simulink model "PubIfDecisionLSM_MDL"  (R2020b)
settings: configuration reference "DspaceConfig" (kept outside this file)
PostLoadFcn:
  | if any(exist('dsrtsu_mdlpostloadfcn', 'file') ~= 0), dsrtsu_mdlpostloadfcn('Execute', bdroot); end
InitFcn:
  | , if any(exist('rtifpga_mdlclblib', 'file') ~= 0), rtifpga_mdlclblib('Init', bdroot); end,
  | , if any(exist('dsmpb_private', 'file') ~= 0), dsmpb_private('dsmpb_mdlclblib', 'Init', bdroot); end,
values from neighbouring files (symbols this model uses):
  P_LSM_ALC_Enable = 0.0    [LSM_Parameter.sldd]
  P_LSM_AwayEdge_offset = 0.1    [LSM_Parameter.sldd]
  P_LSM_CentValidErr = 1.0    [LSM_Parameter.sldd]
  P_LSM_DOP_C0_EN_Limit = 0.8    [LSM_Parameter.sldd]
  P_LSM_DOP_C0_out_Limit = 2.0    [LSM_Parameter.sldd]
  P_LSM_DOP_C1_EN_Limit : value not decoded    [LSM_Parameter.sldd]
  P_LSM_DOP_C1_out_Limit : value not decoded    [LSM_Parameter.sldd]
  P_LSM_DOP_C1AndC2_Lim_X : value not decoded    [LSM_Parameter.sldd]
  P_LSM_DOP_C2_EN_Limit : value not decoded    [LSM_Parameter.sldd]
  P_LSM_DOP_C2_out_Limit : value not decoded    [LSM_Parameter.sldd]
  P_LSM_DOP_In_Pre2Dop_Dis = 1.0    [LSM_Parameter.sldd]
  P_LSM_DOP_Out_Pre2Dop_Dis = 2.0    [LSM_Parameter.sldd]
  P_LSM_DOP_PreDis_X : value not decoded    [LSM_Parameter.sldd]
  P_LSM_DOP_PreDis_Y : value not decoded    [LSM_Parameter.sldd]
  P_LSM_DOPEnableSW = 1.0    [LSM_Parameter.sldd]
  P_LSM_DOPValid_CheckTime = 0.06    [LSM_Parameter.sldd]
  P_LSM_DoubleLine_Curr2Cent_Dislimit = 0.5    [LSM_Parameter.sldd]
  P_LSM_DoubleLine_Dop2Cent_Dislimit = 0.5    [LSM_Parameter.sldd]
  P_LSM_DoubleLine_DOPOut_C1 : value not decoded    [LSM_Parameter.sldd]
  P_LSM_DoubleLine_Pre2Cent_Dislimit = 1.0    [LSM_Parameter.sldd]
  P_LSM_Error_Limit = 0.5    [LSM_Parameter.sldd]
  P_LSM_IFV2CenterAxis = 0.0    [LSM_Parameter.sldd]
  P_LSM_IFV2RearAxis = 0.0    [LSM_Parameter.sldd]
  P_LSM_Line2Edge_limit = 0.5    [LSM_Parameter.sldd]
  P_LSM_Line_Error = 0.1    [LSM_Parameter.sldd]
  P_LSM_LineSTD_Limit = 0.15    [LSM_Parameter.sldd]
  P_LSM_NOH_Switch = 0.0    [LSM_Parameter.sldd]
  P_LSM_OTL_C0_Factor = 1.0    [LSM_Parameter.sldd]
  P_LSM_OTL_C1_Factor = 0.5    [LSM_Parameter.sldd]
  P_LSM_OTL_C2_Factor = 0.5    [LSM_Parameter.sldd]
  P_LSM_Pre2OnlyLineDis = 5.0    [LSM_Parameter.sldd]
  P_LSM_Pre_t = 0.0    [LSM_Parameter.sldd]
  P_LSM_SingleLine_Cent2Edge_Dislimit = 100.0    [LSM_Parameter.sldd]
  P_LSM_SingleLine_Curr2Cent_Dislimit = 0.2    [LSM_Parameter.sldd]
  P_LSM_SingleLine_Dop2Cent_Dislimit = 0.2    [LSM_Parameter.sldd]
  P_LSM_SingleLine_DOPOut_C1 : value not decoded    [LSM_Parameter.sldd]
  P_LSM_SingleLine_Pre2Cent_Dislimit = 0.5    [LSM_Parameter.sldd]
  P_LSM_TJALimitSpd = 60.0    [LSM_Parameter.sldd]
undefined symbols (not defined in the file or in its folder): P_lCS_IFV2CenterAxis, P_LCS_IFV2RearAxis, P_LSM_EntryEdge_offset, P_LSM_EntryLnChngEnSwitch, P_LSM_EntryVanishDis, P_LSM_LinetLostTime, P_LSM_LineWijCal_C12, P_LSM_LineWijCal_C13, P_LSM_MapValid_ErrorSwitch, P_LSM_PosLineLcFac, P_LSM_SpdLim_Stub_Spd, P_LSM_SpdLim_StubLength, P_LSM_SpdTurnAlarm
libraries: simulink x324, TrueDurationTime x11
(part 2 of 25)

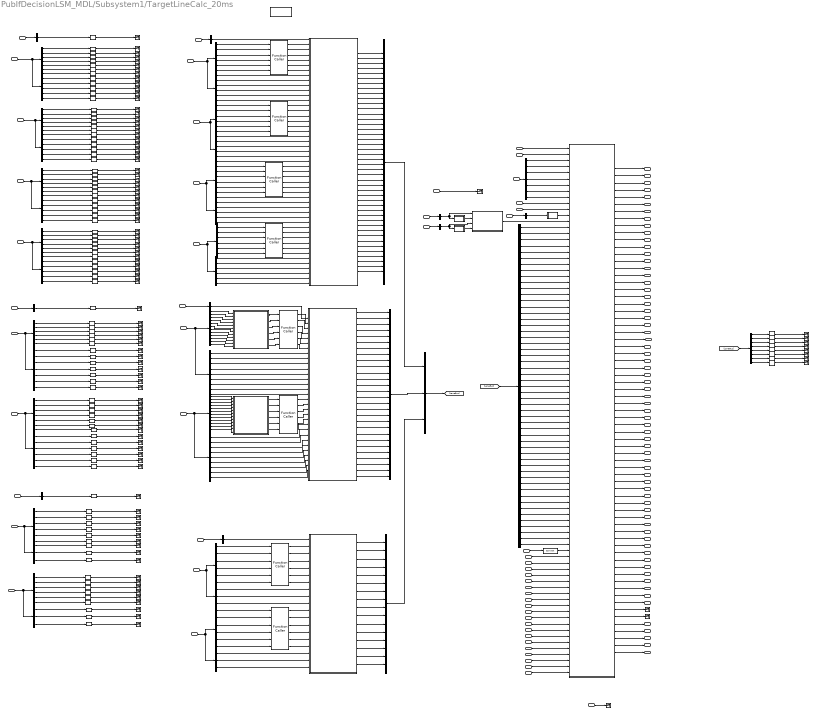
== system PubIfDecisionLSM_MDL/Subsystem1/TargetLineCalc_20ms ==
  vRef : Inport
  kap : Inport  Port=2
  EQ4_LA_ELEM_0 : Inport  Port=3
  EQ4_LA_ELEM_1 : Inport  Port=4
  EQ4_LA_ELEM_2 : Inport  Port=5
  EQ4_LA_ELEM_3 : Inport  Port=6
  LA_HDR : Inport  Port=7
  EQ4_LH_ELEM_0 : Inport  Port=8
  EQ4_LH_ELEM_1 : Inport  Port=9
  LH_HDR : Inport  Port=10
  EQ4_LRE_ELEM : Inport  Port=11
  EQ4_LRE_ELEM1 : Inport  Port=12
  LRE_HDR : Inport  Port=13
  P0TargetLine : Inport  Port=14  OutDataTypeStr=Bus: TOS_P0_TARGET_LINE_BUS
  ACCMode : Inport  Port=15
  HWASts : Inport  Port=16
  ESSSts : Inport  Port=17
  LCKSts : Inport  Port=18
  pathPredValid : Inport  Port=19
  pathPredC3 : Inport  Port=20
  pathPredC2 : Inport  Port=21
  pathPredC1 : Inport  Port=22
  pathPredC0 : Inport  Port=23
  pathPredCnt : Inport  Port=24
  PLAN_ALC_Decision : Inport  Port=25
  RFM_INTERSEC_ALERT : Inport  Port=26
  RFM_ROAD : Inport  Port=27  OutDataTypeStr=Bus: RFM_ROAD_BUS  PortDimensions=1  BusOutputAsStruct=on
  RFM_CURRENT_LANE : Inport  Port=28
  RFM_RIGHT_LANE : Inport  Port=29
  RFM_BRANCH : Inport  Port=30
  RFM_LINE_ENTRY_CL : Inport  Port=31
  RFM_LINE_EXIT_CL : Inport  Port=32
  RFM_LINE_CL : Inport  Port=33
  RFM_TSR_BUS : Inport  Port=34
  RFM_REC_LANES : Inport  Port=35
  RFM_LINE_L1 : Inport  Port=36
  RFM_LINE_R1 : Inport  Port=37
  RFM_LINE_L2 : Inport  Port=38
  RFM_LINE_R2 : Inport  Port=39
  Bus Creator : BusCreator  Inputs=44
  Bus Creator1 : BusCreator  Inputs=28
  Bus Creator2 : BusCreator  Inputs=16
  Bus Creator3 : BusCreator  Inputs=3
  Bus Selector{,1..3,25..26,32..33} (8 alike) : BusSelector  OutputSignals=LA_Line_C0,LA_Line_C1,LA_Line_C2,LA_Line_C3,LA_View_Range_Start,LA_View_Range_End
  Bus Selector10 : BusSelector  OutputSignals=LH.LeftLaneChange,LH.RightLaneChange,LA.L1Conf,LH.LH1Conf,LH.LH2Conf,LA.L4Conf,LA.L1C3,LH.LH1C3,LH.LH2C3,LA.L4C3,LA.L1C2,LH.LH1C2,LH.LH2C2,LA.L4C2,LA.L1C1,LH.LH1C1,LH.LH2C1,LA.L4C1,LA.L1C0,LH.LH1C0,LH.LH2C0,LA.L4C0,LA.L1DxMax,LH.LH1DxMax,LH.LH2DxMax,LA.L4DxMax,LA.L1Reliable,LH.LH1Reliable,LH.LH2Reliable,LA.L4Reliable,LRE.LRE1DxMax,LRE.LRE2DxMax,LRE.LRE1C3,LRE.LRE2C3,LRE.LRE1C2,LRE.LRE2C2,LRE.LRE1C1,LRE.LRE2C1,LRE.LRE1C0,LRE.LRE2C0,LRE.LRE1Conf,LRE.LRE2Conf,LRE.LRE1Reliable,LRE.LRE2Reliable,LH.LH1Type,LH.LH2Type,LH.LH1DLM,LH.LH2DLM,LH.LH1Color,LH.LH2Color,LH.LH1DECEL,LH.LH2DECEL,LA.L1Type
  Bus Selector{11..14,27..30} (8 alike) : BusSelector  OutputSignals=LA_Availability_State,LA_Lanemark_Type,LA_DLM_Type,LA_Line_Side,LA_Marker_Width,LA_Confidence
  Bus Selector15 : BusSelector  OutputSignals=LH_Availability_State,LH_Lanemark_Type,LH_DLM_Type,LH_Side,LH_Marker_Width,LH_Crossing,LH_Confidence,LH_Color,LH_DECEL_Type
  Bus Selector16 : BusSelector  OutputSignals=LH_Availability_State,LH_Lanemark_Type,LH_DLM_Type,LH_Side,LH_Marker_Width,LH_Crossing,LH_Confidence,LH_Color,LH_DECEL_Type
  Bus Selector{17..18,39..40} (4 alike) : BusSelector  OutputSignals=LRE_Availability_State,LRE_Side,LRE_Confidence
  Bus Selector19 : BusSelector  OutputSignals=LA_Adjacent_Count
  Bus Selector20 : BusSelector  OutputSignals=LA_Sync_ID
  Bus Selector21 : BusSelector  OutputSignals=LH_Sync_ID
  Bus Selector22 : BusSelector  OutputSignals=LRE_Sync_ID
  Bus Selector23 : BusSelector  OutputSignals=LH_Lanes_Count
  Bus Selector24 : BusSelector  OutputSignals=LRE_Count
  Bus Selector31 : BusSelector  OutputSignals=LA_Adjacent_Count
  Bus Selector34 : BusSelector  OutputSignals=LH_Availability_State,LH_Lanemark_Type,LH_DLM_Type,LH_Side,LH_Marker_Width,LH_Crossing,LH_Confidence
  Bus Selector35 : BusSelector  OutputSignals=LH_Availability_State,LH_Lanemark_Type,LH_DLM_Type,LH_Side,LH_Marker_Width,LH_Crossing,LH_Confidence
  Bus Selector36 : BusSelector  OutputSignals=LH_Lanes_Count
  Bus Selector37 : BusSelector  OutputSignals=LH_Line_First_C0,LH_Line_First_C1,LH_Line_First_C2,LH_Line_First_C3,LH_First_VR_Start,LH_First_VR_End
  Bus Selector38 : BusSelector  OutputSignals=LH_Line_First_C0,LH_Line_First_C1,LH_Line_First_C2,LH_Line_First_C3,LH_First_VR_Start,LH_First_VR_End
  Bus Selector4 : BusSelector  OutputSignals=LH_Line_First_C0,LH_Line_First_C1,LH_Line_First_C2,LH_Line_First_C3,LH_First_VR_Start,LH_First_VR_End,LH_Line_Second_C0,LH_Line_Second_C1,LH_Line_Second_C2,LH_Line_Second_C3,LH_Second_VR_Start,LH_Second_VR_End
  Bus Selector41 : BusSelector  OutputSignals=LRE_Count
  Bus Selector{6..7,42..43} (4 alike) : BusSelector  OutputSignals=LRE_Line_C0,LRE_Line_C1,LRE_Line_C2,LRE_Line_C3,LRE_View_Range_Start,LRE_View_Range_End
  Bus Selector5 : BusSelector  OutputSignals=LH_Line_First_C0,LH_Line_First_C1,LH_Line_First_C2,LH_Line_First_C3,LH_First_VR_Start,LH_First_VR_End,LH_Line_Second_C0,LH_Line_Second_C1,LH_Line_Second_C2,LH_Line_Second_C3,LH_Second_VR_Start,LH_Second_VR_End
  Bus Selector8 : BusSelector  OutputSignals=OTL_Valid,OTL_C3,OTL_C2,OTL_C1,OTL_C0,OTL_Range,OTL_Cnt
  Bus Selector9 : BusSelector  OutputSignals=LA.L1Conf,LA.L1DxMax,LH.LH1Conf,LH.LH1DxMax,LH.LH2Conf,LH.LH2C3,LA.L4Conf,LA.L4DxMax
  Data Type Conversion : DataTypeConversion
  DetectChange : Subsystem
  DetectChange1 : Subsystem
  DetectChange2 : Subsystem
  EQ4_LA_ELEM_4 : InportShadow  Port=3
  EQ4_LA_ELEM_5 : InportShadow  Port=4
  EQ4_LA_ELEM_6 : InportShadow  Port=5
  EQ4_LA_ELEM_7 : InportShadow  Port=6
  EQ4_LH_ELEM_2 : InportShadow  Port=9
  EQ4_LH_ELEM_3 : InportShadow  Port=8
  EQ4_LRE_ELEM2 : InportShadow  Port=12
  EQ4_LRE_ELEM3 : InportShadow  Port=11
  Function Caller{,1..7} (8 alike) : FunctionCaller  FunctionPrototype=[a0,a1,a2,a3,Rmin,Rmax] = f(A0,A1,A2,A3,Range_min,Range_max)  InputArgumentSpecifications=<Enter example>  OutputArgumentSpecifications=<Enter example>
  LALine : MATLAB Function  TreatAsAtomicUnit=on
  LA_HDR1 : InportShadow  Port=7
  LA_HDR2 : InportShadow  Port=7
  LHLine : MATLAB Function  TreatAsAtomicUnit=on
  LHLine1 : MATLAB Function  TreatAsAtomicUnit=on
  LHLine2 : MATLAB Function  TreatAsAtomicUnit=on
  LH_HDR1 : InportShadow  Port=10
  LH_HDR2 : InportShadow  Port=10
  LRELine : MATLAB Function  TreatAsAtomicUnit=on
  LRE_HDR1 : InportShadow  Port=13
  LRE_HDR2 : InportShadow  Port=13
  MATLAB Function : MATLAB Function  TreatAsAtomicUnit=on
  Signal Copy{,1..101,103} (103 alike) : SignalConversion  OverrideOpt=off
  Simulink Function : Subsystem  TreatAsAtomicUnit=on
  TargetLineCalc : Subsystem
  Terminator{,1..106} (107 alike) : Terminator
  TJALineValid : Outport
  TJALineC3 : Outport  Port=2
  TJALineC2 : Outport  Port=3
  TJALineC1 : Outport  Port=4
  TJALineC0 : Outport  Port=5
  TJARange : Outport  Port=6
  LCKLineValid : Outport  Port=7
  LCKLineC3 : Outport  Port=8
  LCKLineC2 : Outport  Port=9
  LCKLineC1 : Outport  Port=10
  LCKLineC0 : Outport  Port=11
  LCKRange : Outport  Port=12
  HWALineValid : Outport  Port=13
  HWALineC3 : Outport  Port=14
  HWALineC2 : Outport  Port=15
  HWALineC1 : Outport  Port=16
  HWALineC0 : Outport  Port=17
  HWARange : Outport  Port=18
  HWALeLineValid : Outport  Port=19
  HWALeLineC3 : Outport  Port=20
  HWALeLineC2 : Outport  Port=21
  HWALeLineC1 : Outport  Port=22
  HWALeLineC0 : Outport  Port=23
  HWALeRange : Outport  Port=24
  HWARiLineRValid : Outport  Port=25
  HWARiLineC3 : Outport  Port=26
  HWARiLineC2 : Outport  Port=27
  HWARiLineC1 : Outport  Port=28
  HWARiLineC0 : Outport  Port=29
  HWARiRange : Outport  Port=30
  SingleLineLost_b : Outport  Port=31
  DoubleLineLost_b : Outport  Port=32
  dyDiff : Outport  Port=33
  HeadAngDiff : Outport  Port=34
  MLeLane : Outport  Port=35
  RoadWidth : Outport  Port=36
  LeftLaneChange : Outport  Port=37
  RightLaneChange : Outport  Port=38
  MRiLane : Outport  Port=39
  MrcStopLane : Outport  Port=40
  HWALeLineVirtual : Outport  Port=41
  HWARiLineVirtual : Outport  Port=42
  LeLineLcAvailable : Outport  Port=43
  RiLineLcAvailable : Outport  Port=44
  ESSLineValid : Outport  Port=45
  ESSLineC3 : Outport  Port=46
  ESSLineC2 : Outport  Port=47
  ESSLineC1 : Outport  Port=48
  ESSLineC0 : Outport  Port=49
  ESSRange : Outport  Port=50
  ESSLeLineValid : Outport  Port=51
  ESSLeLineC3 : Outport  Port=52
  ESSLeLineC2 : Outport  Port=53
  ESSLeLineC1 : Outport  Port=54
  ESSLeLineC0 : Outport  Port=55
  ESSLeRange : Outport  Port=56
  ESSRiLineValid : Outport  Port=57
  ESSRiLineC3 : Outport  Port=58
  ESSRiLineC2 : Outport  Port=59
  ESSRiLineC1 : Outport  Port=60
  ESSRiLineC0 : Outport  Port=61
  ESSRiRange : Outport  Port=62
  PilotSts : Outport  Port=63
  PilotTurnSwSts : Outport  Port=64
  PilotSPLDist : Outport  Port=65
  PilotSPL : Outport  Port=66
  TJALineSource : Outport  Port=67
  wires:
  TargetLineCalc/40(MrcStopLane) -> MrcStopLane/1
  TargetLineCalc/39(MRiLane) -> MRiLane/1  "MRiLane"
  kap/1 -> TargetLineCalc/1(kap)
  vRef/1 -> TargetLineCalc/2(vRef)
  P0TargetLine/1 -> Bus Selector8/1
  Bus Selector8/2 -> TargetLineCalc/4(aOTL)  "<OTL_C3>"
  Bus Selector8/3 -> TargetLineCalc/5(bOTL)  "<OTL_C2>"
  Bus Selector8/1 -> TargetLineCalc/3(OTLineValid)  "<OTL_Valid>"
  Bus Selector8/4 -> TargetLineCalc/6(cOTL)  "<OTL_C1>"
  Bus Selector8/5 -> TargetLineCalc/7(dOTL)  "<OTL_C0>"
  Bus Selector8/6 -> TargetLineCalc/8(dxMax)  "<OTL_Range>"
  Bus Selector8/7 -> TargetLineCalc/9(OTLCount)  "<OTL_Cnt>"
  ACCMode/1 -> TargetLineCalc/10(ACCMode)
  HWASts/1 -> TargetLineCalc/11(HWASts)
  pathPredC2/1 -> TargetLineCalc/69(pathPredC2)
  pathPredC1/1 -> TargetLineCalc/70(pathPredC1)
  pathPredC3/1 -> TargetLineCalc/68(pathPredC3)
  pathPredValid/1 -> Data Type Conversion/1
  ESSSts/1 -> TargetLineCalc/72(ESSSts)
  pathPredC0/1 -> TargetLineCalc/71(pathPredC0)
  pathPredCnt/1 -> Terminator1/1
  Data Type Conversion/1 -> TargetLineCalc/67(pathPredValid)
  Bus Selector2/5 -> Function Caller2/5  "<LA_View_Range_Start>"
  Function Caller6/4 -> LRELine/5(LRE1A3)
  Function Caller6/2 -> LRELine/3(LRE1A1)
  Function Caller6/1 -> LRELine/2(LRE1A0)
  Bus Selector1/6 -> Function Caller1/6  "<LA_View_Range_End>"
  Function Caller6/6 -> LRELine/7(LRE1RaMax)  "Rmax"
  Bus Selector6/5 -> Function Caller6/5  "<LRE_View_Range_Start>"
  EQ4_LA_ELEM_0/1 -> Bus Selector11/1, Bus Selector/1
  EQ4_LA_ELEM_2/1 -> Bus Selector13/1, Bus Selector2/1
  EQ4_LRE_ELEM/1 -> Bus Selector17/1, Bus Selector6/1
  Function Caller6/5 -> LRELine/6(LRE1RaMin)  "Rmin"
  EQ4_LRE_ELEM1/1 -> Bus Selector18/1, Bus Selector7/1
  Bus Selector6/6 -> Function Caller6/6  "<LRE_View_Range_End>"
  Bus Creator2/1 -> Bus Creator3/3  "LRE"
  Function Caller7/6 -> LRELine/16(LRE2RaMax)  "Rmax"
  Function Caller2/5 -> LALine/30(L3RaMin)  "Rmin"
  Bus Selector7/6 -> Function Caller7/6  "<LRE_View_Range_End>"
  Bus Selector7/5 -> Function Caller7/5  "<LRE_View_Range_Start>"
  Function Caller7/5 -> LRELine/15(LRE2RaMin)  "Rmin"
  Function Caller7/3 -> LRELine/13(LRE2A2)
  Bus Selector1/5 -> Function Caller1/5  "<LA_View_Range_Start>"
  Bus Selector6/1 -> Function Caller6/1  "<LRE_Line_C0>"
  Bus Selector/1 -> Function Caller/1  "<LA_Line_C0>"
  Function Caller3/4 -> LALine/41(L4A3)
  Function Caller7/1 -> LRELine/11(LRE2A0)
  Bus Selector2/4 -> Function Caller2/4  "<LA_Line_C3>"
  Function Caller3/1 -> LALine/38(L4A0)
  Bus Creator/1 -> Bus Creator3/1  "LA"
  Bus Selector3/2 -> Function Caller3/2  "<LA_Line_C1>"
  Bus Selector3/3 -> Function Caller3/3  "<LA_Line_C2>"
  Bus Selector3/4 -> Function Caller3/4  "<LA_Line_C3>"
  Bus Selector/3 -> Function Caller/3  "<LA_Line_C2>"
  Function Caller2/3 -> LALine/28(L3A2)
  Bus Selector/4 -> Function Caller/4  "<LA_Line_C3>"
  Function Caller1/3 -> LALine/16(L2A2)
  Function Caller1/5 -> LALine/18(L2RaMin)  "Rmin"
  Function Caller/3 -> LALine/4(L1A2)  "A2"
  Bus Selector2/3 -> Function Caller2/3  "<LA_Line_C2>"
  Bus Selector1/3 -> Function Caller1/3  "<LA_Line_C2>"
  Function Caller7/4 -> LRELine/14(LRE2A3)
  Bus Selector1/2 -> Function Caller1/2  "<LA_Line_C1>"
  Function Caller3/2 -> LALine/39(L4A1)
  Bus Selector1/1 -> Function Caller1/1  "<LA_Line_C0>"
  Bus Selector7/4 -> Function Caller7/4  "<LRE_Line_C3>"
  Bus Selector2/1 -> Function Caller2/1  "<LA_Line_C0>"
  Bus Selector3/6 -> Function Caller3/6  "<LA_View_Range_End>"
  Function Caller/6 -> LALine/7(L1RaMax)  "Rmax"
  Function Caller1/2 -> LALine/15(L2A1)
  Bus Selector7/2 -> Function Caller7/2  "<LRE_Line_C1>"
  Bus Selector2/2 -> Function Caller2/2  "<LA_Line_C1>"
  Bus Selector2/6 -> Function Caller2/6  "<LA_View_Range_End>"
  Function Caller1/1 -> LALine/14(L2A0)
  Function Caller/4 -> LALine/5(L1A3)  "A3"
  Bus Selector3/5 -> Function Caller3/5  "<LA_View_Range_Start>"
  Bus Selector7/1 -> Function Caller7/1  "<LRE_Line_C0>"
  Function Caller/2 -> LALine/3(L1A1)  "A1"
  Function Caller6/3 -> LRELine/4(LRE1A2)
  Bus Selector1/4 -> Function Caller1/4  "<LA_Line_C3>"
  Function Caller1/6 -> LALine/19(L2RaMax)  "Rmax"
  Bus Selector/6 -> Function Caller/6  "<LA_View_Range_End>"
  Function Caller3/6 -> LALine/43(L4RaMax)  "Rmax"
  Function Caller2/1 -> LALine/26(L3A0)
  Function Caller3/5 -> LALine/42(L4RaMin)  "Rmin"
  Function Caller2/4 -> LALine/29(L3A3)
  Function Caller7/2 -> LRELine/12(LRE2A1)
  Function Caller3/3 -> LALine/40(L4A2)
  Bus Selector7/3 -> Function Caller7/3  "<LRE_Line_C2>"
  EQ4_LA_ELEM_3/1 -> Bus Selector14/1, Bus Selector3/1
  Function Caller/5 -> LALine/6(L1RaMin)  "Rmin"
  Bus Selector/5 -> Function Caller/5  "<LA_View_Range_Start>"
  Bus Selector6/3 -> Function Caller6/3  "<LRE_Line_C2>"
  Function Caller/1 -> LALine/2(L1A0)  "A0"
  Bus Selector6/2 -> Function Caller6/2  "<LRE_Line_C1>"
  Bus Selector6/4 -> Function Caller6/4  "<LRE_Line_C3>"
  Bus Selector3/1 -> Function Caller3/1  "<LA_Line_C0>"
  Bus Creator3/1 -> [LaneBus]
  Function Caller1/4 -> LALine/17(L2A3)
  Bus Selector/2 -> Function Caller/2  "<LA_Line_C1>"
  Function Caller2/2 -> LALine/27(L3A1)
  Function Caller2/6 -> LALine/31(L3RaMax)  "Rmax"
  EQ4_LA_ELEM_1/1 -> Bus Selector12/1, Bus Selector1/1
  Bus Selector11/1 -> LALine/8(L1Avail)  "<LA_Availability_State>"
  Bus Selector11/2 -> LALine/9(L1LineType)  "<LA_Lanemark_Type>"
  Bus Selector11/3 -> LALine/10(L1DLType)  "<LA_DLM_Type>"
  Bus Selector11/4 -> LALine/11(L1SideType)  "<LA_Line_Side>"
  Bus Selector11/5 -> LALine/12(L1Wid)  "<LA_Marker_Width>"
  Bus Selector12/1 -> LALine/20(L2Avail)  "<LA_Availability_State>"
  Bus Selector12/2 -> LALine/21(L2LineType)  "<LA_Lanemark_Type>"
  Bus Selector12/3 -> LALine/22(L2DLType)  "<LA_DLM_Type>"
  Bus Selector12/4 -> LALine/23(L2SideType)  "<LA_Line_Side>"
  Bus Selector12/5 -> LALine/24(L2Wid)  "<LA_Marker_Width>"
  Bus Selector13/1 -> LALine/32(L3Avail)  "<LA_Availability_State>"
  Bus Selector13/2 -> LALine/33(L3LineType)  "<LA_Lanemark_Type>"
  Bus Selector13/3 -> LALine/34(L3DLType)  "<LA_DLM_Type>"
  Bus Selector13/4 -> LALine/35(L3SideType)  "<LA_Line_Side>"
  Bus Selector13/5 -> LALine/36(L3Wid)  "<LA_Marker_Width>"
  Bus Selector14/1 -> LALine/44(L4Avail)  "<LA_Availability_State>"
  Bus Selector14/2 -> LALine/45(L4LineType)  "<LA_Lanemark_Type>"
  Bus Selector14/3 -> LALine/46(L4DLType)  "<LA_DLM_Type>"
  Bus Selector14/4 -> LALine/47(L4SideType)  "<LA_Line_Side>"
  Bus Selector14/5 -> LALine/48(L4Wid)  "<LA_Marker_Width>"
  Bus Selector17/1 -> LRELine/8(LRE1Avail)  "<LRE_Availability_State>"
  Bus Selector17/2 -> LRELine/9(LRE1SideType)  "<LRE_Side>"
  Bus Selector18/1 -> LRELine/17(LRE2Avail)  "<LRE_Availability_State>"
  Bus Selector18/2 -> LRELine/18(LRE2SideType)  "<LRE_Side>"
  LA_HDR/1 -> Bus Selector19/1
  LA_HDR1/1 -> Bus Selector20/1
  LH_HDR1/1 -> Bus Selector21/1
  LRE_HDR1/1 -> Bus Selector22/1
  Bus Selector20/1 -> DetectChange1/1(In1), MATLAB Function/1(LA_Sync_ID)  "<LA_Sync_ID>"
  Bus Selector21/1 -> DetectChange2/1(In1), MATLAB Function/3(LH_Sync_ID)  "<LH_Sync_ID>"
  Bus Selector22/1 -> DetectChange/1(In1)  "<LRE_Sync_ID>"
  LRE_HDR/1 -> Bus Selector24/1
  Bus Selector24/1 -> LRELine/1(LRE_Count)  "<LRE_Count>"
  Bus Selector19/1 -> LALine/1(LA_Count)  "<LA_Adjacent_Count>"
  DetectChange/1(Out1) -> TargetLineCalc/12(LRELineUpdate)
  DetectChange1/1(Out1) -> MATLAB Function/2(LA_Update)
  DetectChange2/1(Out1) -> MATLAB Function/4(LH_Upadate)
  TargetLineCalc/1(TJALineValid) -> TJALineValid/1  "TJALineValid"
  TargetLineCalc/2(TJALineA3) -> TJALineC3/1  "TJALineC3"
  TargetLineCalc/3(TJALineA2) -> TJALineC2/1  "TJALineC2"
  TargetLineCalc/4(TJALineA1) -> TJALineC1/1  "TJALineC1"
  TargetLineCalc/5(TJALineA0) -> TJALineC0/1  "TJALineC0"
  TargetLineCalc/6(TJALineRange) -> TJARange/1  "TJARange"
  TargetLineCalc/7(LCKLineValid) -> LCKLineValid/1  "LCKLineValid"
  TargetLineCalc/8(LCKLineA3) -> LCKLineC3/1  "LCKLineC3"
  TargetLineCalc/9(LCKLineA2) -> LCKLineC2/1  "LCKLineC2"
  TargetLineCalc/10(LCKLineA1) -> LCKLineC1/1  "LCKLineC1"
  TargetLineCalc/11(LCKLineA0) -> LCKLineC0/1  "LCKLineC0"
  TargetLineCalc/12(LCKLineRange) -> LCKRange/1  "LCKRange"
  TargetLineCalc/13(HWALineValid) -> HWALineValid/1
  TargetLineCalc/14(HWALineA3) -> HWALineC3/1
  TargetLineCalc/15(HWALineA2) -> HWALineC2/1
  TargetLineCalc/16(HWALineA1) -> HWALineC1/1
  TargetLineCalc/17(HWALineA0) -> HWALineC0/1
  TargetLineCalc/18(HWALineRange) -> HWARange/1
  TargetLineCalc/19(HWALineLValid1) -> HWALeLineValid/1
  TargetLineCalc/20(HWALineLA3) -> HWALeLineC3/1
  TargetLineCalc/21(HWALineLA2) -> HWALeLineC2/1
  TargetLineCalc/22(HWALineLA1) -> HWALeLineC1/1
  TargetLineCalc/23(HWALineLA0) -> HWALeLineC0/1
  TargetLineCalc/24(HWALineLRange) -> HWALeRange/1
  TargetLineCalc/25(HWALineRValid) -> HWARiLineRValid/1
  TargetLineCalc/26(HWALineRA3) -> HWARiLineC3/1
  TargetLineCalc/27(HWALineRA2) -> HWARiLineC2/1
  TargetLineCalc/28(HWALineRA1) -> HWARiLineC1/1
  TargetLineCalc/29(HWALineRA0) -> HWARiLineC0/1
  TargetLineCalc/30(HWALineRRange0) -> HWARiRange/1
  TargetLineCalc/33(MLeLane) -> MLeLane/1  "MLeLane"
  TargetLineCalc/34(RoadWidth) -> RoadWidth/1
  TargetLineCalc/35(SingleLineLost_b) -> SingleLineLost_b/1
  TargetLineCalc/36(DoubleLineLost_b) -> DoubleLineLost_b/1
  TargetLineCalc/45(ESSLineValid) -> ESSLineValid/1  "ESSLineValid"
  TargetLineCalc/46(ESSLineA3) -> ESSLineC3/1  "ESSLineC3"
  TargetLineCalc/47(ESSLineA2) -> ESSLineC2/1  "ESSLineC2"
  TargetLineCalc/48(ESSLineA1) -> ESSLineC1/1  "ESSLineC1"
  TargetLineCalc/49(ESSLineA0) -> ESSLineC0/1  "ESSLineC0"
  TargetLineCalc/50(ESSLineRange) -> ESSRange/1  "ESSRange"
  TargetLineCalc/51(ESSLineLValid) -> ESSLeLineValid/1  "ESSLeLineValid"
  TargetLineCalc/52(ESSLineLA3) -> ESSLeLineC3/1  "ESSLeLineC3"
  TargetLineCalc/53(ESSLineLA2) -> ESSLeLineC2/1  "ESSLeLineC2"
  TargetLineCalc/54(ESSLineLA1) -> ESSLeLineC1/1  "ESSLeLineC1"
  TargetLineCalc/55(ESSLineLA0) -> ESSLeLineC0/1  "ESSLeLineC0"
  TargetLineCalc/56(ESSLineLRange) -> ESSLeRange/1  "ESSLeRange"
  TargetLineCalc/57(ESSLineRValid) -> ESSRiLineValid/1  "ESSRiLineValid"
  TargetLineCalc/58(ESSLineRA3) -> ESSRiLineC3/1  "ESSRiLineC3"
  TargetLineCalc/59(ESSLineRA2) -> ESSRiLineC2/1  "ESSRiLineC2"
  TargetLineCalc/60(ESSLineRA1) -> ESSRiLineC1/1  "ESSRiLineC1"
  TargetLineCalc/61(ESSLineRA0) -> ESSRiLineC0/1  "ESSRiLineC0"
  TargetLineCalc/62(ESSLineRRange) -> ESSRiRange/1  "ESSRiRange"
  TargetLineCalc/63(ESSLineLock_b) -> Terminator2/1
  TargetLineCalc/64(leftLaneCurise_b) -> Terminator/1
  MATLAB Function/1(y) -> TargetLineCalc/13(LALineUpdate)
  PLAN_ALC_Decision/1 -> Terminator4/1
  TargetLineCalc/37(LeLineCrossing) -> LeftLaneChange/1  "LeLineCrossing"
  TargetLineCalc/38(RiLineCrossing) -> RightLaneChange/1  "RiLineCrossing"
  Bus Selector11/6 -> LALine/13(L1Confidence)  "<LA_Confidence>"
  Bus Selector14/6 -> LALine/49(L4Confidence)  "<LA_Confidence>"
  Bus Selector12/6 -> LALine/25(L2Confidence)  "<LA_Confidence>"
  Bus Selector13/6 -> LALine/37(L3Confidence)  "<LA_Confidence>"
  LALine/28(L3DxMin) -> Bus Creator/28
  LALine/27(L3C3) -> Bus Creator/27
  LALine/29(L3DxMax) -> Bus Creator/29
  LALine/26(L3C2) -> Bus Creator/26
  LALine/30(L3Type) -> Bus Creator/30
  LALine/25(L3C1) -> Bus Creator/25
  LALine/31(L3DLM) -> Bus Creator/31
  LALine/24(L3C0) -> Bus Creator/24
  LALine/32(L3Width) -> Bus Creator/32
  LALine/23(L3Conf) -> Bus Creator/23
  LALine/33(L3Reliable) -> Bus Creator/33
  LALine/22(L2Reliable) -> Bus Creator/22
  LALine/34(L4Conf) -> Bus Creator/34
  LALine/21(L2Width) -> Bus Creator/21
  LALine/35(L4C0) -> Bus Creator/35
  LALine/20(L2DLM) -> Bus Creator/20
  LALine/36(L4C1) -> Bus Creator/36
  LALine/19(L2Type) -> Bus Creator/19
  LALine/37(L4C2) -> Bus Creator/37
  LALine/18(L2DxMax) -> Bus Creator/18
  LALine/38(L4C3) -> Bus Creator/38
  LALine/17(L2DxMin) -> Bus Creator/17
  LALine/39(L4DxMin) -> Bus Creator/39
  LALine/16(L2C3) -> Bus Creator/16
  LALine/40(L4DxMax) -> Bus Creator/40
  LALine/15(L2C2) -> Bus Creator/15
  LALine/41(L4Type) -> Bus Creator/41
  LALine/14(L2C1) -> Bus Creator/14
  LALine/42(L4DLM) -> Bus Creator/42
  LALine/13(L2C0) -> Bus Creator/13
  LALine/43(L4Width) -> Bus Creator/43
  LALine/12(L2Conf) -> Bus Creator/12
  LALine/44(L4Reliable) -> Bus Creator/44
  LALine/11(L1Reliable) -> Bus Creator/11
  LALine/10(L1Width) -> Bus Creator/10
  LALine/9(L1DLM) -> Bus Creator/9
  LALine/8(L1Type) -> Bus Creator/8
  LALine/7(L1DxMax) -> Bus Creator/7
  LALine/6(L1DxMin) -> Bus Creator/6
  LALine/5(L1C3) -> Bus Creator/5
  LALine/4(L1C2) -> Bus Creator/4
  LALine/3(L1C1) -> Bus Creator/3
  LALine/2(L1C0) -> Bus Creator/2
  LALine/1(L1Conf) -> Bus Creator/1
  LRELine/9(LRE2Conf) -> Bus Creator2/9
  LRELine/8(LRE1Reliable) -> Bus Creator2/8
  LRELine/10(LRE2C0) -> Bus Creator2/10
  LRELine/7(LRE1DxMax) -> Bus Creator2/7
  LRELine/11(LRE2C1) -> Bus Creator2/11
  LRELine/6(LRE1DxMin) -> Bus Creator2/6
  LRELine/12(LRE2C2) -> Bus Creator2/12
  LRELine/5(LRE1C3) -> Bus Creator2/5
  LRELine/13(LRE2C3) -> Bus Creator2/13
  LRELine/4(LRE1C2) -> Bus Creator2/4
  LRELine/14(LRE2DxMin) -> Bus Creator2/14
  LRELine/3(LRE1C1) -> Bus Creator2/3
  LRELine/15(LRE2DxMax) -> Bus Creator2/15
  LRELine/2(LRE1C0) -> Bus Creator2/2
  LRELine/16(LRE2Reliable) -> Bus Creator2/16
  LRELine/1(LRE1Conf) -> Bus Creator2/1
  Bus Selector17/3 -> LRELine/10(LRE1Confdience)  "<LRE_Confidence>"
  Bus Selector18/3 -> LRELine/19(LRE2Confdience)  "<LRE_Confidence>"
  TargetLineCalc/65(PilotSts) -> PilotSts/1
  TargetLineCalc/31(pre_dy_Error) -> dyDiff/1
  TargetLineCalc/32(pre_HeadAng_Error) -> HeadAngDiff/1
  RFM_INTERSEC_ALERT/1 -> TargetLineCalc/74(RFM_INTERSEC_ALERT)
  RFM_ROAD/1 -> TargetLineCalc/78(RFM_ROAD)
  RFM_CURRENT_LANE/1 -> TargetLineCalc/75(RFM_CURRENT_LANE)
  TargetLineCalc/66(PilotTurnSwSts) -> PilotTurnSwSts/1
  RFM_LINE_ENTRY_CL/1 -> TargetLineCalc/79(RFM_LINE_ENTRY_CL)
  RFM_LINE_EXIT_CL/1 -> TargetLineCalc/80(RFM_LINE_EXIT_CL)
  TargetLineCalc/67(PilotSPLDist) -> PilotSPLDist/1
  TargetLineCalc/68(PilotSPL) -> PilotSPL/1
  [LaneBus] -> Bus Selector9/1
  Bus Selector9/1 -> Signal Copy/1  "<L1Conf>"
  Bus Selector9/2 -> Signal Copy1/1  "<L1DxMax>"
  Bus Selector9/3 -> Signal Copy2/1  "<LH1Conf>"
  Bus Selector9/4 -> Signal Copy3/1  "<LH1DxMax>"
  Bus Selector9/5 -> Signal Copy4/1  "<LH2Conf>"
  Bus Selector9/6 -> Signal Copy5/1  "<LH2C3>"
  Bus Selector9/7 -> Signal Copy6/1  "<L4Conf>"
  Bus Selector9/8 -> Signal Copy7/1  "<L4DxMax>"
  Signal Copy/1 -> Terminator3/1  "LSM_L1_Conf"
  Signal Copy1/1 -> Terminator5/1  "LSM_L1_Range"
  Signal Copy2/1 -> Terminator6/1  "LSM_L2_Conf"
  Signal Copy3/1 -> Terminator7/1  "LSM_L2_Range"
  Signal Copy4/1 -> Terminator8/1  "LSM_L3_Conf"
  Signal Copy5/1 -> Terminator9/1  "LSM_L3_Range"
  Signal Copy6/1 -> Terminator10/1  "LSM_L4_Conf"
  Signal Copy7/1 -> Terminator11/1  "LSM_L4_Range"
  Bus Selector29/6 -> Signal Copy41/1  "<LA_Confidence>"
  Bus Selector28/6 -> Signal Copy30/1  "<LA_Confidence>"
  Bus Selector30/6 -> Signal Copy54/1  "<LA_Confidence>"
  Bus Selector27/6 -> Signal Copy20/1  "<LA_Confidence>"
  Bus Selector31/1 -> Signal Copy8/1  "<LA_Adjacent_Count>"
  LA_HDR2/1 -> Bus Selector31/1
  Bus Selector30/5 -> Signal Copy56/1  "<LA_Marker_Width>"
  Bus Selector30/4 -> Signal Copy55/1  "<LA_Line_Side>"
  Bus Selector30/3 -> Signal Copy53/1  "<LA_DLM_Type>"
  Bus Selector30/2 -> Signal Copy52/1  "<LA_Lanemark_Type>"
  Bus Selector30/1 -> Signal Copy51/1  "<LA_Availability_State>"
  Bus Selector29/5 -> Signal Copy44/1  "<LA_Marker_Width>"
  Bus Selector29/4 -> Signal Copy43/1  "<LA_Line_Side>"
  Bus Selector29/3 -> Signal Copy42/1  "<LA_DLM_Type>"
  Bus Selector29/2 -> Signal Copy40/1  "<LA_Lanemark_Type>"
  Bus Selector29/1 -> Signal Copy39/1  "<LA_Availability_State>"
  Bus Selector28/5 -> Signal Copy32/1  "<LA_Marker_Width>"
  Bus Selector28/4 -> Signal Copy31/1  "<LA_Line_Side>"
  Bus Selector28/3 -> Signal Copy29/1  "<LA_DLM_Type>"
  Bus Selector28/2 -> Signal Copy28/1  "<LA_Lanemark_Type>"
  Bus Selector28/1 -> Signal Copy27/1  "<LA_Availability_State>"
  Bus Selector27/5 -> Signal Copy19/1  "<LA_Marker_Width>"
  Bus Selector27/4 -> Signal Copy18/1  "<LA_Line_Side>"
  Bus Selector27/3 -> Signal Copy17/1  "<LA_DLM_Type>"
  Bus Selector27/2 -> Signal Copy16/1  "<LA_Lanemark_Type>"
  Bus Selector27/1 -> Signal Copy15/1  "<LA_Availability_State>"
  EQ4_LA_ELEM_5/1 -> Bus Selector26/1, Bus Selector28/1
  Bus Selector25/2 -> Signal Copy10/1  "<LA_Line_C1>"
  Bus Selector33/1 -> Signal Copy45/1  "<LA_Line_C0>"
  Bus Selector25/5 -> Signal Copy13/1  "<LA_View_Range_Start>"
  EQ4_LA_ELEM_7/1 -> Bus Selector33/1, Bus Selector30/1
  Bus Selector25/6 -> Signal Copy14/1  "<LA_View_Range_End>"
  Bus Selector26/4 -> Signal Copy24/1  "<LA_Line_C3>"
  Bus Selector33/5 -> Signal Copy49/1  "<LA_View_Range_Start>"
  Bus Selector32/6 -> Signal Copy38/1  "<LA_View_Range_End>"
  Bus Selector32/2 -> Signal Copy34/1  "<LA_Line_C1>"
  Bus Selector33/6 -> Signal Copy50/1  "<LA_View_Range_End>"
  Bus Selector32/1 -> Signal Copy33/1  "<LA_Line_C0>"
  Bus Selector26/1 -> Signal Copy21/1  "<LA_Line_C0>"
  Bus Selector26/2 -> Signal Copy22/1  "<LA_Line_C1>"
  Bus Selector26/3 -> Signal Copy23/1  "<LA_Line_C2>"
  Bus Selector32/3 -> Signal Copy35/1  "<LA_Line_C2>"
  Bus Selector25/4 -> Signal Copy12/1  "<LA_Line_C3>"
  Bus Selector25/3 -> Signal Copy11/1  "<LA_Line_C2>"
  Bus Selector33/4 -> Signal Copy48/1  "<LA_Line_C3>"
  Bus Selector33/3 -> Signal Copy47/1  "<LA_Line_C2>"
  Bus Selector33/2 -> Signal Copy46/1  "<LA_Line_C1>"
  Bus Selector32/4 -> Signal Copy36/1  "<LA_Line_C3>"
  Bus Selector25/1 -> Signal Copy9/1  "<LA_Line_C0>"
  Bus Selector26/5 -> Signal Copy25/1  "<LA_View_Range_Start>"
  EQ4_LA_ELEM_6/1 -> Bus Selector32/1, Bus Selector29/1
  EQ4_LA_ELEM_4/1 -> Bus Selector25/1, Bus Selector27/1
  Bus Selector26/6 -> Signal Copy26/1  "<LA_View_Range_End>"
  Bus Selector32/5 -> Signal Copy37/1  "<LA_View_Range_Start>"
  Signal Copy8/1 -> Terminator12/1  "LSM_LA_Adjacent_Count"
  Signal Copy15/1 -> Terminator19/1  "LSM_LA_ELEM_0_Availability_State"
  Signal Copy16/1 -> Terminator20/1  "LSM_LA_ELEM_0_Lanemark_Type"
  Signal Copy17/1 -> Terminator21/1  "LSM_LA_ELEM_0_DLM_Type"
  Signal Copy18/1 -> Terminator22/1  "LSM_LA_ELEM_0_Line_Side"
  Signal Copy19/1 -> Terminator24/1  "LSM_LA_ELEM_0_Marker_Width"
  Signal Copy20/1 -> Terminator23/1  "LSM_LA_ELEM_0_Confidence"
  Signal Copy27/1 -> Terminator31/1  "LSM_LA_ELEM_1_Availability_State"
  Signal Copy28/1 -> Terminator32/1  "LSM_LA_ELEM_1_Lanemark_Type"
  Signal Copy31/1 -> Terminator34/1  "LSM_LA_ELEM_1_Line_Side"
  Signal Copy32/1 -> Terminator36/1  "LSM_LA_ELEM_1_Marker_Width"
  Signal Copy30/1 -> Terminator35/1  "LSM_LA_ELEM_1_Confidence"
  Signal Copy29/1 -> Terminator33/1  "LSM_LA_ELEM_1_DLM_Type"
  Signal Copy39/1 -> Terminator43/1  "LSM_LA_ELEM_2_Availability_State"
  Signal Copy40/1 -> Terminator44/1  "LSM_LA_ELEM_2_Lanemark_Type"
  Signal Copy44/1 -> Terminator48/1  "LSM_LA_ELEM_2_Marker_Width"
  Signal Copy43/1 -> Terminator46/1  "LSM_LA_ELEM_2_Line_Side"
  Signal Copy41/1 -> Terminator47/1  "LSM_LA_ELEM_2_Confidence"
  Signal Copy42/1 -> Terminator45/1  "LSM_LA_ELEM_2_DLM_Type"
  Signal Copy51/1 -> Terminator55/1  "LSM_LA_ELEM_3_Availability_State"
  Signal Copy52/1 -> Terminator56/1  "LSM_LA_ELEM_3_Lanemark_Type"
  Signal Copy55/1 -> Terminator58/1  "LSM_LA_ELEM_3_Line_Side"
  Signal Copy56/1 -> Terminator60/1  "LSM_LA_ELEM_3_Marker_Width"
  Signal Copy54/1 -> Terminator59/1  "LSM_LA_ELEM_3_Confidence"
  Signal Copy53/1 -> Terminator57/1  "LSM_LA_ELEM_3_DLM_Type"
  Signal Copy9/1 -> Terminator13/1  "LSM_LA_ELEM_0_C0"
  Signal Copy10/1 -> Terminator14/1  "LSM_LA_ELEM_0_C1"
  Signal Copy11/1 -> Terminator15/1  "LSM_LA_ELEM_0_C2"
  Signal Copy12/1 -> Terminator16/1  "LSM_LA_ELEM_0_C3"
  Signal Copy13/1 -> Terminator17/1  "LSM_LA_ELEM_0_Range_Start"
  Signal Copy14/1 -> Terminator18/1  "LSM_LA_ELEM_0_Range_End"
  Signal Copy26/1 -> Terminator30/1  "LSM_LA_ELEM_1_Range_End"
  Signal Copy25/1 -> Terminator29/1  "LSM_LA_ELEM_1_Range_Start"
  Signal Copy24/1 -> Terminator28/1  "LSM_LA_ELEM_1_C3"
  Signal Copy23/1 -> Terminator27/1  "LSM_LA_ELEM_1_C2"
  Signal Copy22/1 -> Terminator26/1  "LSM_LA_ELEM_1_C1"
  Signal Copy21/1 -> Terminator25/1  "LSM_LA_ELEM_1_C0"
  Signal Copy50/1 -> Terminator54/1  "LSM_LA_ELEM_3_Range_End"
  Signal Copy49/1 -> Terminator53/1  "LSM_LA_ELEM_3_Range_Start"
  Signal Copy48/1 -> Terminator52/1  "LSM_LA_ELEM_3_C3"
  Signal Copy47/1 -> Terminator51/1  "LSM_LA_ELEM_3_C2"
  Signal Copy46/1 -> Terminator50/1  "LSM_LA_ELEM_3_C1"
  Signal Copy45/1 -> Terminator49/1  "LSM_LA_ELEM_3_C0"
  Signal Copy38/1 -> Terminator42/1  "LSM_LA_ELEM_2_Range_End"
  Signal Copy37/1 -> Terminator41/1  "LSM_LA_ELEM_2_Range_Start"
  Signal Copy36/1 -> Terminator40/1  "LSM_LA_ELEM_2_C3"
  Signal Copy35/1 -> Terminator39/1  "LSM_LA_ELEM_2_C2"
  Signal Copy34/1 -> Terminator38/1  "LSM_LA_ELEM_2_C1"
  Signal Copy33/1 -> Terminator37/1  "LSM_LA_ELEM_2_C0"
  Bus Selector35/7 -> Signal Copy74/1  "<LH_Confidence>"
  Bus Selector34/7 -> Signal Copy61/1  "<LH_Confidence>"
  Bus Selector35/6 -> Signal Copy82/1  "<LH_Crossing>"
  Bus Selector34/6 -> Signal Copy69/1  "<LH_Crossing>"
  Bus Selector36/1 -> Signal Copy57/1  "<LH_Lanes_Count>"
  LH_HDR2/1 -> Bus Selector36/1
  Bus Selector35/5 -> Signal Copy80/1  "<LH_Marker_Width>"
  Bus Selector35/4 -> Signal Copy81/1  "<LH_Side>"
  Bus Selector35/3 -> Signal Copy79/1  "<LH_DLM_Type>"
  Bus Selector35/2 -> Signal Copy78/1  "<LH_Lanemark_Type>"
  Bus Selector35/1 -> Signal Copy77/1  "<LH_Availability_State>"
  Bus Selector34/4 -> Signal Copy68/1  "<LH_Side>"
  Bus Selector34/3 -> Signal Copy66/1  "<LH_DLM_Type>"
  Bus Selector34/2 -> Signal Copy65/1  "<LH_Lanemark_Type>"
  Bus Selector34/1 -> Signal Copy64/1  "<LH_Availability_State>"
  Bus Selector34/5 -> Signal Copy67/1  "<LH_Marker_Width>"
  Bus Selector38/6 -> Signal Copy83/1  "<LH_First_VR_End>"
  Bus Selector37/5 -> Signal Copy70/1  "<LH_First_VR_Start>"
  Bus Selector37/1 -> Signal Copy58/1  "<LH_Line_First_C0>"
  Bus Selector37/6 -> Signal Copy63/1  "<LH_First_VR_End>"
  Bus Selector37/2 -> Signal Copy59/1  "<LH_Line_First_C1>"
  EQ4_LH_ELEM_2/1 -> Bus Selector38/1, Bus Selector35/1
  Bus Selector38/2 -> Signal Copy72/1  "<LH_Line_First_C1>"
  Bus Selector37/4 -> Signal Copy62/1  "<LH_Line_First_C3>"
  EQ4_LH_ELEM_3/1 -> Bus Selector37/1, Bus Selector34/1
  Bus Selector38/3 -> Signal Copy73/1  "<LH_Line_First_C2>"
  Bus Selector38/4 -> Signal Copy75/1  "<LH_Line_First_C3>"
  Bus Selector38/1 -> Signal Copy71/1  "<LH_Line_First_C0>"
  Bus Selector37/3 -> Signal Copy60/1  "<LH_Line_First_C2>"
  Bus Selector38/5 -> Signal Copy76/1  "<LH_First_VR_Start>"
  Bus Selector40/3 -> Signal Copy94/1  "<LRE_Confidence>"
  Bus Selector39/3 -> Signal Copy93/1  "<LRE_Confidence>"
  Bus Selector41/1 -> Signal Copy84/1  "<LRE_Count>"
  LRE_HDR2/1 -> Bus Selector41/1
  Bus Selector40/2 -> Signal Copy100/1  "<LRE_Side>"
  Bus Selector40/1 -> Signal Copy98/1  "<LRE_Availability_State>"
  Bus Selector39/2 -> Signal Copy85/1  "<LRE_Side>"
  Bus Selector39/1 -> Signal Copy91/1  "<LRE_Availability_State>"
  Bus Selector42/4 -> Signal Copy88/1  "<LRE_Line_C3>"
  Bus Selector42/2 -> Signal Copy86/1  "<LRE_Line_C1>"
  Bus Selector42/3 -> Signal Copy87/1  "<LRE_Line_C2>"
  Bus Selector43/3 -> Signal Copy96/1  "<LRE_Line_C2>"
  Bus Selector43/1 -> Signal Copy101/1  "<LRE_Line_C0>"
  Bus Selector43/2 -> Signal Copy95/1  "<LRE_Line_C1>"
  Bus Selector43/4 -> Signal Copy97/1  "<LRE_Line_C3>"
  Bus Selector42/1 -> Signal Copy92/1  "<LRE_Line_C0>"
  Bus Selector43/5 -> Signal Copy103/1  "<LRE_View_Range_Start>"
  Bus Selector43/6 -> Signal Copy99/1  "<LRE_View_Range_End>"
  Bus Selector42/6 -> Signal Copy89/1  "<LRE_View_Range_End>"
  EQ4_LRE_ELEM2/1 -> Bus Selector43/1, Bus Selector40/1
  EQ4_LRE_ELEM3/1 -> Bus Selector42/1, Bus Selector39/1
  Bus Selector42/5 -> Signal Copy90/1  "<LRE_View_Range_Start>"
  Signal Copy57/1 -> Terminator67/1  "LSM_LH_Count"
  Signal Copy64/1 -> Terminator65/1  "LSM_LH_ELEM_0_Availability_State"
  Signal Copy65/1 -> Terminator66/1  "LSM_LH_ELEM_0_Lanemark_Type"
  Signal Copy67/1 -> Terminator70/1  "LSM_LH_ELEM_0_Marker_Width"
  Signal Copy69/1 -> Terminator72/1  "LSM_LH_ELEM_0_Crossing"
  Signal Copy68/1 -> Terminator69/1  "LSM_LH_ELEM_0_Line_Side"
  Signal Copy66/1 -> Terminator68/1  "LSM_LH_ELEM_0_DLM_Type"
  Signal Copy61/1 -> Terminator71/1  "LSM_LH_ELEM_0_Confidence"
  Signal Copy77/1 -> Terminator79/1  "LSM_LH_ELEM_1_Availability_State"
  Signal Copy74/1 -> Terminator84/1  "LSM_LH_ELEM_1_Confidence"
  Signal Copy79/1 -> Terminator81/1  "LSM_LH_ELEM_1_DLM_Type"
  Signal Copy80/1 -> Terminator83/1  "LSM_LH_ELEM_1_Marker_Width"
  Signal Copy78/1 -> Terminator80/1  "LSM_LH_ELEM_1_Lanemark_Type"
  Signal Copy81/1 -> Terminator82/1  "LSM_LH_ELEM_1_Line_Side"
  Signal Copy82/1 -> Terminator85/1  "LSM_LH_ELEM_1_Crossing"
  Signal Copy85/1 -> Terminator98/1  "LSM_LRE_ELEM_0_Line_Side"
  Signal Copy91/1 -> Terminator96/1  "LSM_LRE_ELEM_0_Availability_State"
  Signal Copy93/1 -> Terminator97/1  "LSM_LRE_ELEM_0_Confidence"
  Signal Copy98/1 -> Terminator104/1  "LSM_LRE_ELEM_1_Availability_State"
  Signal Copy100/1 -> Terminator106/1  "LSM_LRE_ELEM_1_Line_Side"
  Signal Copy94/1 -> Terminator105/1  "LSM_LRE_ELEM_1_Confidence"
  Signal Copy63/1 -> Terminator64/1  "LSM_LH_ELEM_0_VR_End"
  Signal Copy70/1 -> Terminator63/1  "LSM_LH_ELEM_0_VR_Start"
  Signal Copy62/1 -> Terminator62/1  "LSM_LH_ELEM_0_C3"
  Signal Copy60/1 -> Terminator61/1  "LSM_LH_ELEM_0_C2"
  Signal Copy58/1 -> Terminator73/1  "LSM_LH_ELEM_0_C0"
  Signal Copy59/1 -> Terminator74/1  "LSM_LH_ELEM_0_C1"
  Signal Copy83/1 -> Terminator78/1  "LSM_LH_ELEM_1_VR_End"
  Signal Copy76/1 -> Terminator77/1  "LSM_LH_ELEM_1_VR_Start"
  Signal Copy75/1 -> Terminator76/1  "LSM_LH_ELEM_1_C3"
  Signal Copy73/1 -> Terminator75/1  "LSM_LH_ELEM_1_C2"
  Signal Copy72/1 -> Terminator87/1  "LSM_LH_ELEM_1_C1"
  Signal Copy71/1 -> Terminator86/1  "LSM_LH_ELEM_1_C0"
  Signal Copy89/1 -> Terminator95/1  "LSM_LRE_ELEM_0_Range_End"
  Signal Copy90/1 -> Terminator94/1  "LSM_LRE_ELEM_0_Range_Start"
  Signal Copy88/1 -> Terminator93/1  "LSM_LRE_ELEM_0_C3"
  Signal Copy87/1 -> Terminator92/1  "LSM_LRE_ELEM_0_C2"
  Signal Copy86/1 -> Terminator91/1  "LSM_LRE_ELEM_0_C1"
  Signal Copy92/1 -> Terminator90/1  "LSM_LRE_ELEM_0_C0"
  Signal Copy84/1 -> Terminator99/1  "LSM_LRE_Count"
  Signal Copy99/1 -> Terminator103/1  "LSM_LRE_ELEM_1_Range_End"
  Signal Copy103/1 -> Terminator102/1  "LSM_LRE_ELEM_1_Range_Start"
  Signal Copy97/1 -> Terminator101/1  "LSM_LRE_ELEM_1_C3"
  Signal Copy96/1 -> Terminator100/1  "LSM_LRE_ELEM_1_C2"
  Signal Copy95/1 -> Terminator89/1  "LSM_LRE_ELEM_1_C1"
  Signal Copy101/1 -> Terminator88/1  "LSM_LRE_ELEM_1_C0"
  LCKSts/1 -> TargetLineCalc/73(LCKSts)
  Bus Selector10/1 -> TargetLineCalc/14(LeftLine_Change)  "<LeftLaneChange>"
  Bus Selector10/3 -> TargetLineCalc/16(L1_Conf)  "<L1Conf>"
  Bus Selector10/4 -> TargetLineCalc/17(L2_Conf)  "<LH1Conf>"
  Bus Selector10/5 -> TargetLineCalc/18(L3_Conf)  "<LH2Conf>"
  Bus Selector10/6 -> TargetLineCalc/19(L4_Conf)  "<L4Conf>"
  Bus Selector10/7 -> TargetLineCalc/20(L1_A3)  "<L1C3>"
  Bus Selector10/8 -> TargetLineCalc/21(L2_A3)  "<LH1C3>"
  Bus Selector10/10 -> TargetLineCalc/23(L4_A3)  "<L4C3>"
  Bus Selector10/11 -> TargetLineCalc/24(L1_A2)  "<L1C2>"
  Bus Selector10/12 -> TargetLineCalc/25(L2_A2)  "<LH1C2>"
  Bus Selector10/14 -> TargetLineCalc/27(L4_A2)  "<L4C2>"
  Bus Selector10/15 -> TargetLineCalc/28(L1_A1)  "<L1C1>"
  Bus Selector10/16 -> TargetLineCalc/29(L2_A1)  "<LH1C1>"
  Bus Selector10/18 -> TargetLineCalc/31(L4_A1)  "<L4C1>"
  Bus Selector10/19 -> TargetLineCalc/32(L1_A0)  "<L1C0>"
  Bus Selector10/20 -> TargetLineCalc/33(L2_A0)  "<LH1C0>"
  Bus Selector10/22 -> TargetLineCalc/35(L4_A0)  "<L4C0>"
  Bus Selector10/23 -> TargetLineCalc/36(L1_R)  "<L1DxMax>"
  Bus Selector10/24 -> TargetLineCalc/37(L2_R)  "<LH1DxMax>"
  Bus Selector10/26 -> TargetLineCalc/39(L4_R)  "<L4DxMax>"
  Bus Selector10/27 -> TargetLineCalc/40(L1_Re)  "<L1Reliable>"
  Bus Selector10/28 -> TargetLineCalc/41(L2_Re)  "<LH1Reliable>"
  Bus Selector10/30 -> TargetLineCalc/43(L4_Re)  "<L4Reliable>"
  Bus Selector10/31 -> TargetLineCalc/44(Edge1_R)  "<LRE1DxMax>"
  Bus Selector10/32 -> TargetLineCalc/45(Edge2_R)  "<LRE2DxMax>"
  Bus Selector10/33 -> TargetLineCalc/46(Edge1_A3)  "<LRE1C3>"
  Bus Selector10/34 -> TargetLineCalc/47(Edge2_A3)  "<LRE2C3>"
  Bus Selector10/35 -> TargetLineCalc/48(Edge1_A2)  "<LRE1C2>"
  Bus Selector10/36 -> TargetLineCalc/49(Edge2_A2)  "<LRE2C2>"
  Bus Selector10/37 -> TargetLineCalc/50(Edge1_A1)  "<LRE1C1>"
  Bus Selector10/38 -> TargetLineCalc/51(Edge2_A1)  "<LRE2C1>"
  Bus Selector10/39 -> TargetLineCalc/52(Edge1_A0)  "<LRE1C0>"
  Bus Selector10/40 -> TargetLineCalc/53(Edge2_A0)  "<LRE2C0>"
  Bus Selector10/41 -> TargetLineCalc/54(Edge1_Conf)  "<LRE1Conf>"
  Bus Selector10/42 -> TargetLineCalc/55(Edge2_Conf)  "<LRE2Conf>"
  Bus Selector10/43 -> TargetLineCalc/56(Edge1_Re)  "<LRE1Reliable>"
  Bus Selector10/44 -> TargetLineCalc/57(Edge2_Re)  "<LRE2Reliable>"
  Bus Selector10/45 -> TargetLineCalc/58(LeftLineType)  "<LH1Type>"
  Bus Selector10/47 -> TargetLineCalc/60(LeftDLM)  "<LH1DLM>"
  Bus Selector10/49 -> TargetLineCalc/62(LH1Color)  "<LH1Color>"
  RFM_TSR_BUS/1 -> TargetLineCalc/82(RFM_TSR_BUS)
  TargetLineCalc/69(TJALineSource) -> TJALineSource/1
  RFM_REC_LANES/1 -> TargetLineCalc/83(RFM_REC_LANES)
  RFM_RIGHT_LANE/1 -> TargetLineCalc/76(RFM_RIGHT_LANE)
  RFM_BRANCH/1 -> TargetLineCalc/77(RFM_BRANCH)
  RFM_LINE_L1/1 -> TargetLineCalc/84(RFM_LINE_L1)
  RFM_LINE_R1/1 -> TargetLineCalc/85(RFM_LINE_R1)
  RFM_LINE_L2/1 -> TargetLineCalc/86(RFM_LINE_L2)
  RFM_LINE_R2/1 -> TargetLineCalc/87(RFM_LINE_R2)
  RFM_LINE_CL/1 -> TargetLineCalc/81(RFM_LINE_CL)
  [LaneBus] -> Bus Selector10/1
  Bus Selector5/6 -> LHLine2/6(LHRaMax)  "<LH_First_VR_End>"
  Bus Selector5/4 -> LHLine2/4(LHA3)  "<LH_Line_First_C3>"
  LHLine/19(LH2C3) -> Bus Creator1/19
  Bus Selector15/5 -> LHLine/12(LH1Wid)  "<LH_Marker_Width>"
  LHLine/26(RightLaneChange) -> Bus Creator1/26
  Bus Selector5/1 -> LHLine2/1(LHA0)  "<LH_Line_First_C0>"
  LHLine/20(LH2DxMin) -> Bus Creator1/20
  Bus Selector16/8 -> LHLine/30(LH2_Color)  "<LH_Color>"
  Bus Selector15/7 -> LHLine/14(LH1Confidence)  "<LH_Confidence>"
  Bus Selector4/3 -> LHLine1/3(LHA2)  "<LH_Line_First_C2>"
  LHLine/22(LH2Type) -> Bus Creator1/22
  Function Caller4/4 -> LHLine/5(LH1A3)
  Function Caller4/1 -> LHLine/2(LH1A0)
  Bus Selector15/1 -> LHLine/8(LH1Avail)  "<LH_Availability_State>"
  LHLine/3(LH1C1) -> Bus Creator1/3
  Bus Selector5/8 -> LHLine2/8(LH_ELEM_Second_C1)  "<LH_Line_Second_C1>"
  LHLine/13(LH1Color) -> Bus Creator1/13
  LHLine/7(LH1DxMax) -> Bus Creator1/7
  LHLine2/3(LHC2) -> Function Caller5/3
  Bus Selector16/2 -> LHLine/24(LH2LineType)  "<LH_Lanemark_Type>"
  Bus Selector4/2 -> LHLine1/2(LHA1)  "<LH_Line_First_C1>"
  Bus Selector16/3 -> LHLine/25(LH2DLType)  "<LH_DLM_Type>"
  Bus Selector4/6 -> LHLine1/6(LHRaMax)  "<LH_First_VR_End>"
  LHLine/17(LH2C1) -> Bus Creator1/17
  LHLine2/2(LHC1) -> Function Caller5/2
  LHLine/11(LH1Reliable) -> Bus Creator1/11
  Bus Selector5/10 -> LHLine2/10(LH_ELEM_Second_C3)  "<LH_Line_Second_C3>"
  Bus Selector5/9 -> LHLine2/9(LH_ELEM_Second_C2)  "<LH_Line_Second_C2>"
  Function Caller4/6 -> LHLine/7(LH1RaMax)  "Rmax"
  Function Caller5/4 -> LHLine/20(LH2A3)
  Bus Creator1/1 -> Bus Creator3/2  "LH"
  LHLine/25(LH2Reliable) -> Bus Creator1/25
  LHLine/4(LH1C2) -> Bus Creator1/4
  Bus Selector5/3 -> LHLine2/3(LHA2)  "<LH_Line_First_C2>"
  Bus Selector4/7 -> LHLine1/7(LH_ELEM_Second_C0)  "<LH_Line_Second_C0>"
  LHLine1/6(LHDxMax) -> Function Caller4/6
  LHLine/21(LH2DxMax) -> Bus Creator1/21
  Bus Selector16/7 -> LHLine/29(LH2Confidence)  "<LH_Confidence>"
  Bus Selector4/5 -> LHLine1/5(LHRaMin)  "<LH_First_VR_Start>"
  Bus Selector15/4 -> LHLine/11(LH1SideType)  "<LH_Side>"
  LHLine/8(LH1Type) -> Bus Creator1/8
  LHLine/1(LH1Conf) -> Bus Creator1/1
  LHLine/27(LH2Color) -> Bus Creator1/27
  LHLine/9(LH1DLM) -> Bus Creator1/9
  LHLine/24(LH2Width) -> Bus Creator1/24
  LHLine/23(LH2DLM) -> Bus Creator1/23
  LHLine1/4(LHC3) -> Function Caller4/4
  Bus Selector4/9 -> LHLine1/9(LH_ELEM_Second_C2)  "<LH_Line_Second_C2>"
  Bus Selector5/11 -> LHLine2/11(LH_ELEM_Second_Start)  "<LH_Second_VR_Start>"
  LHLine2/4(LHC3) -> Function Caller5/4
  Bus Selector5/7 -> LHLine2/7(LH_ELEM_Second_C0)  "<LH_Line_Second_C0>"
  LHLine/12(LeftLaneChange) -> Bus Creator1/12
  LHLine/16(LH2C0) -> Bus Creator1/16
  Function Caller5/5 -> LHLine/21(LH2RaMin)  "Rmin"
  LHLine1/3(LHC2) -> Function Caller4/3
  Bus Selector5/12 -> LHLine2/12(LH_ELEM_Second_End)  "<LH_Second_VR_End>"
  LHLine/5(LH1C3) -> Bus Creator1/5
  Bus Selector4/8 -> LHLine1/8(LH_ELEM_Second_C1)  "<LH_Line_Second_C1>"
  LHLine1/2(LHC1) -> Function Caller4/2
  LHLine1/5(LHDxMin) -> Function Caller4/5
  Bus Selector4/11 -> LHLine1/11(LH_ELEM_Second_Start)  "<LH_Second_VR_Start>"
  Function Caller5/3 -> LHLine/19(LH2A2)
  LHLine1/1(LHC0) -> Function Caller4/1
  Bus Selector16/5 -> LHLine/27(LH2Wid)  "<LH_Marker_Width>"
  Bus Selector4/12 -> LHLine1/12(LH_ELEM_Second_End)  "<LH_Second_VR_End>"
  LHLine2/6(LHDxMax) -> Function Caller5/6
  LHLine/2(LH1C0) -> Bus Creator1/2
  LHLine/18(LH2C2) -> Bus Creator1/18
  Bus Selector4/1 -> LHLine1/1(LHA0)  "<LH_Line_First_C0>"
  Bus Selector16/4 -> LHLine/26(LH2SideType)  "<LH_Side>"
  Bus Selector15/2 -> LHLine/9(LH1LineType)  "<LH_Lanemark_Type>"
  Function Caller5/1 -> LHLine/17(LH2A0)
  Function Caller4/2 -> LHLine/3(LH1A1)
  LHLine/6(LH1DxMin) -> Bus Creator1/6
  Bus Selector15/8 -> LHLine/15(LH1_Color)  "<LH_Color>"
  LHLine/10(LH1Width) -> Bus Creator1/10
  LHLine2/1(LHC0) -> Function Caller5/1
  Bus Selector5/5 -> LHLine2/5(LHRaMin)  "<LH_First_VR_Start>"
  LH_HDR/1 -> Bus Selector23/1
  Bus Selector15/6 -> LHLine/13(LH1Crossing)  "<LH_Crossing>"
  Function Caller5/6 -> LHLine/22(LH2RaMax)  "Rmax"
  Function Caller5/2 -> LHLine/18(LH2A1)
  Bus Selector16/1 -> LHLine/23(LH2Avail)  "<LH_Availability_State>"
  Bus Selector4/4 -> LHLine1/4(LHA3)  "<LH_Line_First_C3>"
  LHLine2/5(LHDxMin) -> Function Caller5/5
  Bus Selector4/10 -> LHLine1/10(LH_ELEM_Second_C3)  "<LH_Line_Second_C3>"
  Function Caller4/5 -> LHLine/6(LH1RaMin)  "Rmin"
  Bus Selector5/2 -> LHLine2/2(LHA1)  "<LH_Line_First_C1>"
  EQ4_LH_ELEM_0/1 -> Bus Selector15/1, Bus Selector4/1
  Function Caller4/3 -> LHLine/4(LH1A2)
  LHLine/15(LH2Conf) -> Bus Creator1/15
  EQ4_LH_ELEM_1/1 -> Bus Selector16/1, Bus Selector5/1
  Bus Selector15/3 -> LHLine/10(LH1DLType)  "<LH_DLM_Type>"
  Bus Selector16/6 -> LHLine/28(LH2Crossing)  "<LH_Crossing>"
  Bus Selector23/1 -> LHLine/1(LH_Count)  "<LH_Lanes_Count>"
  Bus Selector15/9 -> LHLine/16(LH1DEType)  "<LH_DECEL_Type>"
  LHLine/14(LH1DECEL) -> Bus Creator1/14
  LHLine/28(LH2DECEL) -> Bus Creator1/28
  Bus Selector16/9 -> LHLine/31(LH2DEType)  "<LH_DECEL_Type>"
  Bus Selector10/2 -> TargetLineCalc/15(RightLine_Change)  "<RightLaneChange>"
  Bus Selector10/9 -> TargetLineCalc/22(L3_A3)  "<LH2C3>"
  Bus Selector10/13 -> TargetLineCalc/26(L3_A2)  "<LH2C2>"
  Bus Selector10/17 -> TargetLineCalc/30(L3_A1)  "<LH2C1>"
  Bus Selector10/21 -> TargetLineCalc/34(L3_A0)  "<LH2C0>"
  Bus Selector10/25 -> TargetLineCalc/38(L3_R)  "<LH2DxMax>"
  Bus Selector10/29 -> TargetLineCalc/42(L3_Re)  "<LH2Reliable>"
  Bus Selector10/46 -> TargetLineCalc/59(RightLineType)  "<LH2Type>"
  Bus Selector10/48 -> TargetLineCalc/61(RightDLM)  "<LH2DLM>"
  Bus Selector10/50 -> TargetLineCalc/63(LH2Color)  "<LH2Color>"
  Bus Selector10/51 -> TargetLineCalc/64(LeftDECELType)  "<LH1DECEL>"
  Bus Selector10/52 -> TargetLineCalc/65(RightDECELType)  "<LH2DECEL>"
  TargetLineCalc/41(HWALeLineVirtual) -> HWALeLineVirtual/1
  TargetLineCalc/42(HWARiLineVirtual) -> HWARiLineVirtual/1
  TargetLineCalc/43(LeLineLcAvailable) -> LeLineLcAvailable/1
  TargetLineCalc/44(RiLineLcAvailable) -> RiLineLcAvailable/1
  Bus Selector10/53 -> TargetLineCalc/66(LLeftType)  "<L1Type>"
